simulink model "model1"  (R2013a)
settings: Solver=ode45  StartTime=0.0  StopTime=10.0  RelTol=1e-3
libraries: fl_lib x40, nesl_utility x2, powerlib x1
settings Model: Creator=hariom  LastModifiedBy=hariom

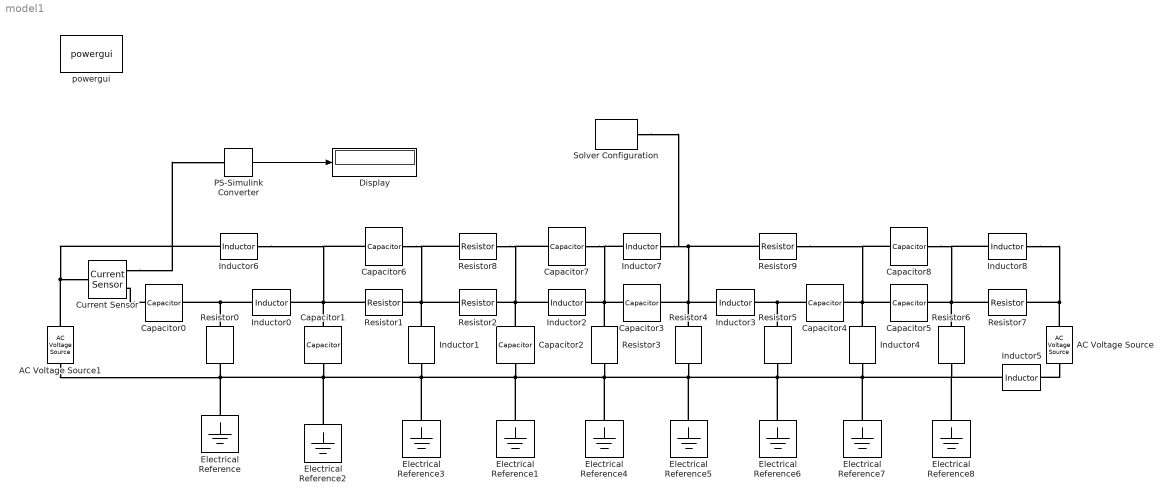
== system model1 ==
  AC Voltage Source : fl_lib/Electrical/Electrical Sources/AC Voltage Source  amp=450 V  shift=0 deg  frequency=50 Hz  omega=0 rad/s  i_Log=off  v_Log=off  LocalVarNames=|i|v  LocalVarDescs=|i|v  LocalVarLogging=[0 0]
  AC Voltage Source1 : fl_lib/Electrical/Electrical Sources/AC Voltage Source  amp=450 V  shift=0 deg  frequency=50 Hz  omega=0 rad/s  i_Log=off  v_Log=off  LocalVarNames=|i|v  LocalVarDescs=|i|v  LocalVarLogging=[0 0]
  Capacitor0 : fl_lib/Electrical/Electrical Elements/Capacitor  c=225 uF  v0=0 V  r=0 Ohm  g=0 1/Ohm  i_Log=off  v_Log=off  vc_Log=off  LocalVarNames=|i|v|vc  LocalVarDescs=|i|v|Internal variable for voltage across capacitor term  LocalVarLogging=[0 0 0]
  Capacitor1 : fl_lib/Electrical/Electrical Elements/Capacitor  c=767 uF  v0=0 V  r=0 Ohm  g=0 1/Ohm  i_Log=off  v_Log=off  vc_Log=off  LocalVarNames=|i|v|vc  LocalVarDescs=|i|v|Internal variable for voltage across capacitor term  LocalVarLogging=[0 0 0]
  Capacitor2 : fl_lib/Electrical/Electrical Elements/Capacitor  c=543 uF  v0=0 V  r=0 Ohm  g=0 1/Ohm  i_Log=off  v_Log=off  vc_Log=off  LocalVarNames=|i|v|vc  LocalVarDescs=|i|v|Internal variable for voltage across capacitor term  LocalVarLogging=[0 0 0]
  Capacitor3 : fl_lib/Electrical/Electrical Elements/Capacitor  c=891 uF  v0=0 V  r=0 Ohm  g=0 1/Ohm  i_Log=off  v_Log=off  vc_Log=off  LocalVarNames=|i|v|vc  LocalVarDescs=|i|v|Internal variable for voltage across capacitor term  LocalVarLogging=[0 0 0]
  Capacitor4 : fl_lib/Electrical/Electrical Elements/Capacitor  c=335 uF  v0=0 V  r=0 Ohm  g=0 1/Ohm  i_Log=off  v_Log=off  vc_Log=off  LocalVarNames=|i|v|vc  LocalVarDescs=|i|v|Internal variable for voltage across capacitor term  LocalVarLogging=[0 0 0]
  Capacitor5 : fl_lib/Electrical/Electrical Elements/Capacitor  c=649 uF  v0=0 V  r=0 Ohm  g=0 1/Ohm  i_Log=off  v_Log=off  vc_Log=off  LocalVarNames=|i|v|vc  LocalVarDescs=|i|v|Internal variable for voltage across capacitor term  LocalVarLogging=[0 0 0]
  Capacitor6 : fl_lib/Electrical/Electrical Elements/Capacitor  c=422 uF  v0=0 V  r=0 Ohm  g=0 1/Ohm  i_Log=off  v_Log=off  vc_Log=off  LocalVarNames=|i|v|vc  LocalVarDescs=|i|v|Internal variable for voltage across capacitor term  LocalVarLogging=[0 0 0]
  Capacitor7 : fl_lib/Electrical/Electrical Elements/Capacitor  c=922 uF  v0=0 V  r=0 Ohm  g=0 1/Ohm  i_Log=off  v_Log=off  vc_Log=off  LocalVarNames=|i|v|vc  LocalVarDescs=|i|v|Internal variable for voltage across capacitor term  LocalVarLogging=[0 0 0]
  Capacitor8 : fl_lib/Electrical/Electrical Elements/Capacitor  c=512 uF  v0=0 V  r=0 Ohm  g=0 1/Ohm  i_Log=off  v_Log=off  vc_Log=off  LocalVarNames=|i|v|vc  LocalVarDescs=|i|v|Internal variable for voltage across capacitor term  LocalVarLogging=[0 0 0]
  Current Sensor : fl_lib/Electrical/Electrical Sensors/Current Sensor  i1_Log=off  v1_Log=off  LocalVarNames=|i1|v1  LocalVarDescs=|i1|v1  LocalVarLogging=[0 0]
  Display : Display
  Electrical Reference{,1..8} (9 alike) : fl_lib/Electrical/Electrical Elements/Electrical Reference  i_Log=off  LocalVarNames=|i  LocalVarDescs=|i  LocalVarLogging=0
  Inductor0 : fl_lib/Electrical/Electrical Elements/Inductor  l=15 mH  i0=0 A  r=0 Ohm  g=1e-9 1/Ohm  i_Log=off  v_Log=off  i_L_Log=off  LocalVarNames=|i|v|i_L  LocalVarDescs=|i|v|Internal variable for current through inductor term  LocalVarLogging=[0 0 0]
  Inductor1 : fl_lib/Electrical/Electrical Elements/Inductor  l=36 mH  i0=0 A  r=0 Ohm  g=1e-9 1/Ohm  i_Log=off  v_Log=off  i_L_Log=off  LocalVarNames=|i|v|i_L  LocalVarDescs=|i|v|Internal variable for current through inductor term  LocalVarLogging=[0 0 0]
  Inductor2 : fl_lib/Electrical/Electrical Elements/Inductor  l=79 mH  i0=0 A  r=0 Ohm  g=1e-9 1/Ohm  i_Log=off  v_Log=off  i_L_Log=off  LocalVarNames=|i|v|i_L  LocalVarDescs=|i|v|Internal variable for current through inductor term  LocalVarLogging=[0 0 0]
  Inductor3 : fl_lib/Electrical/Electrical Elements/Inductor  l=42 mH  i0=0 A  r=0 Ohm  g=1e-9 1/Ohm  i_Log=off  v_Log=off  i_L_Log=off  LocalVarNames=|i|v|i_L  LocalVarDescs=|i|v|Internal variable for current through inductor term  LocalVarLogging=[0 0 0]
  Inductor4 : fl_lib/Electrical/Electrical Elements/Inductor  l=59 mH  i0=0 A  r=0 Ohm  g=1e-9 1/Ohm  i_Log=off  v_Log=off  i_L_Log=off  LocalVarNames=|i|v|i_L  LocalVarDescs=|i|v|Internal variable for current through inductor term  LocalVarLogging=[0 0 0]
  Inductor5 : fl_lib/Electrical/Electrical Elements/Inductor  l=63 mH  i0=0 A  r=0 Ohm  g=1e-9 1/Ohm  i_Log=off  v_Log=off  i_L_Log=off  LocalVarNames=|i|v|i_L  LocalVarDescs=|i|v|Internal variable for current through inductor term  LocalVarLogging=[0 0 0]
  Inductor6 : fl_lib/Electrical/Electrical Elements/Inductor  l=84 mH  i0=0 A  r=0 Ohm  g=1e-9 1/Ohm  i_Log=off  v_Log=off  i_L_Log=off  LocalVarNames=|i|v|i_L  LocalVarDescs=|i|v|Internal variable for current through inductor term  LocalVarLogging=[0 0 0]
  Inductor7 : fl_lib/Electrical/Electrical Elements/Inductor  l=28 mH  i0=0 A  r=0 Ohm  g=1e-9 1/Ohm  i_Log=off  v_Log=off  i_L_Log=off  LocalVarNames=|i|v|i_L  LocalVarDescs=|i|v|Internal variable for current through inductor term  LocalVarLogging=[0 0 0]
  Inductor8 : fl_lib/Electrical/Electrical Elements/Inductor  l=92 mH  i0=0 A  r=0 Ohm  g=1e-9 1/Ohm  i_Log=off  v_Log=off  i_L_Log=off  LocalVarNames=|i|v|i_L  LocalVarDescs=|i|v|Internal variable for current through inductor term  LocalVarLogging=[0 0 0]
  PS-Simulink Converter : nesl_utility/PS-Simulink Converter  PhysicalDomain=network_engine_domain  SubClassName=ps_output  LeftPortType=input  RightPortType=output  PseudoPeriodic=off  Frequencies=[]  Unit=A  AffineConversion=off
  Resistor0 : fl_lib/Electrical/Electrical Elements/Resistor  R=15.25 Ohm  i_Log=off  v_Log=off  LocalVarNames=|i|v  LocalVarDescs=|i|v  LocalVarLogging=[0 0]
  Resistor1 : fl_lib/Electrical/Electrical Elements/Resistor  R=8.69 Ohm  i_Log=off  v_Log=off  LocalVarNames=|i|v  LocalVarDescs=|i|v  LocalVarLogging=[0 0]
  Resistor2 : fl_lib/Electrical/Electrical Elements/Resistor  R=7.43 Ohm  i_Log=off  v_Log=off  LocalVarNames=|i|v  LocalVarDescs=|i|v  LocalVarLogging=[0 0]
  Resistor3 : fl_lib/Electrical/Electrical Elements/Resistor  R=19.79 Ohm  i_Log=off  v_Log=off  LocalVarNames=|i|v  LocalVarDescs=|i|v  LocalVarLogging=[0 0]
  Resistor4 : fl_lib/Electrical/Electrical Elements/Resistor  R=3.85 Ohm  i_Log=off  v_Log=off  LocalVarNames=|i|v  LocalVarDescs=|i|v  LocalVarLogging=[0 0]
  Resistor5 : fl_lib/Electrical/Electrical Elements/Resistor  R=5.91 Ohm  i_Log=off  v_Log=off  LocalVarNames=|i|v  LocalVarDescs=|i|v  LocalVarLogging=[0 0]
  Resistor6 : fl_lib/Electrical/Electrical Elements/Resistor  R=9.53 Ohm  i_Log=off  v_Log=off  LocalVarNames=|i|v  LocalVarDescs=|i|v  LocalVarLogging=[0 0]
  Resistor7 : fl_lib/Electrical/Electrical Elements/Resistor  R=16.76 Ohm  i_Log=off  v_Log=off  LocalVarNames=|i|v  LocalVarDescs=|i|v  LocalVarLogging=[0 0]
  Resistor8 : fl_lib/Electrical/Electrical Elements/Resistor  R=18.04 Ohm  i_Log=off  v_Log=off  LocalVarNames=|i|v  LocalVarDescs=|i|v  LocalVarLogging=[0 0]
  Resistor9 : fl_lib/Electrical/Electrical Elements/Resistor  R=2.12 Ohm  i_Log=off  v_Log=off  LocalVarNames=|i|v  LocalVarDescs=|i|v  LocalVarLogging=[0 0]
  Solver Configuration : nesl_utility/Solver Configuration  PhysicalDomain=network_engine_domain  SubClassName=solver  LeftPortType=input  RightPortType=generic  Accelerate=off  Tones=[]  Harmonics=[]  SimulateNoise=off  Profile=off  UseLocalSampling=off  EnableSwitchedLinearOptims=on  FrequencyDomain=off  UseCCode=off  UseNewInitialization=off  DoDC=off  ResidualTolerance=1e-09  UseLocalSolver=off  LocalSolverChoice=NE_BACKWARD_EULER_ADVANCER  LocalSolverSampleTime=0.001  DoFixedCost=off  MaxNonlinIter=3  MaxModeIter=2  LinearAlgebra=Sparse  DelaysMemoryBudget=1024
  powergui : powerlib/powergui  Priority=1  SimulationMode=Continuous  SolverType=Tustin  SampleTime=50e-6  frequency=60  SPID=off  DisableSnubberDevices=off  DisableRonSwitches=off  DisableVfSwitches=off  SwTol=0  Interpol=off  DisplayEquations=off  frequencyindice=50  Pbase=100e6  ErrMax=1e-4  Iterations=50  UnitsV=kV  UnitsW=MW  FunctionMessages=off  echomessages=off  HookPort=off  EnableUseOfTLC=off  x0status=blocks  RestoreLinks=warning  ResistiveCurrentMeasurement=off  Frange=[0:2:500]  Ylog=off  Xlog=on  ShowGrid=off  save=off  variable=ZData  ZoomFFT=off  StartTime=0.0  cycles=1  DisplayStyle=1  fundamental=60  FreqAxis=off  MaxFrequency=1000  frequencyindicesteady=1  RmsSteady=1  display=off  Ts=0  methode=off
  wires:
  PS-Simulink Converter/1 -> Display/1
  connections:
  Resistor0/LConn1 -- Capacitor0/RConn1 -- Inductor0/LConn1
  Capacitor1/LConn1 -- Inductor6/RConn1 -- Capacitor6/LConn1 -- Resistor1/LConn1 -- Inductor0/RConn1
  Inductor1/LConn1 -- Resistor8/LConn1 -- Capacitor6/RConn1 -- Resistor2/LConn1 -- Resistor1/RConn1
  Capacitor2/LConn1 -- Capacitor7/LConn1 -- Resistor8/RConn1 -- Inductor2/LConn1 -- Resistor2/RConn1
  Resistor3/LConn1 -- Capacitor7/RConn1 -- Inductor7/LConn1 -- Capacitor3/LConn1 -- Inductor2/RConn1
  Resistor4/LConn1 -- Solver Configuration/RConn1 -- Inductor7/RConn1 -- Resistor9/LConn1 -- Capacitor3/RConn1 -- Inductor3/LConn1
  Resistor5/LConn1 -- Inductor3/RConn1 -- Capacitor4/LConn1
  Inductor4/LConn1 -- Capacitor8/LConn1 -- Resistor9/RConn1 -- Capacitor4/RConn1 -- Capacitor5/LConn1
  Resistor6/LConn1 -- Capacitor8/RConn1 -- Inductor8/LConn1 -- Capacitor5/RConn1 -- Resistor7/LConn1
  Inductor8/RConn1 -- AC Voltage Source/LConn1 -- Resistor7/RConn1
  Electrical Reference2/LConn1 -- Electrical Reference3/LConn1 -- Electrical Reference1/LConn1 -- Electrical Reference4/LConn1 -- Electrical Reference5/LConn1 -- Electrical Reference6/LConn1 -- Electrical Reference7/LConn1 -- Electrical Reference8/LConn1 -- Inductor5/RConn1 -- Resistor6/RConn1 -- Inductor4/RConn1 -- Resistor5/RConn1 -- Resistor4/RConn1 -- Resistor3/RConn1 -- Capacitor2/RConn1 -- Inductor1/RConn1 -- Capacitor1/RConn1 -- Electrical Reference/LConn1 -- AC Voltage Source1/RConn1 -- Resistor0/RConn1
  AC Voltage Source/RConn1 -- Inductor5/LConn1
  AC Voltage Source1/LConn1 -- Inductor6/LConn1 -- Current Sensor/LConn1
  Capacitor0/LConn1 -- Current Sensor/RConn2
  Current Sensor/RConn1 -- PS-Simulink Converter/LConn1
